simulink model "PreScan_Vissim_Python_0_2_cs_old"  (R2017b)
settings: Solver=ode5  StartTime=0.0  StopTime=inf  FixedStep=1/200  RelTol=1e-3
PreLoadFcn:
  | mbxruntime.callbacks.PreLoadFcn(bdroot);
PostLoadFcn:
  | mbxruntime.callbacks.PostLoadFcn(bdroot);
InitFcn:
  | mbxruntime.callbacks.InitFcn(bdroot);
StartFcn:
  | mbxruntime.callbacks.StartFcn(bdroot);
StopFcn:
  | mbxruntime.callbacks.StopFcn(bdroot);
model workspace (MAT data in the model file):
  mbox_table : struct (value not decoded)
  model_closed = 0
  sim_status = 0
undefined symbols (not defined in the file or in its folder): DiscIntNeverNeededParam, warningInitialVelocity, x0
libraries: simulink x19, simulink_extras x5, dspnetwork x5, PreScanSimulinkLibrary x4, etargetslib x4
(part 4 of 4)

== system PreScan_Vissim_Python_0_2_cs_old/Toyota_Yaris_Hatchback_1/PathFollower_Preview_1/LateralController/CTRL REFERENCES/Find Reference Point (pref0) on Trajectory closest to P0 Point (p0) ==
  In1 : Inport
  In2 : Inport  Port=2
  In3 : Inport  Port=3
  In4 : Inport  Port=4
  eml_find_closest_trajectory_points0 : MATLAB Function  TreatAsAtomicUnit=on
  Out1 : Outport
  Out2 : Outport  Port=2
  wires:
  eml_find_closest_trajectory_points0/2(Actor_traj_angle) -> Out2/1
  eml_find_closest_trajectory_points0/1(Actor_traj_distance) -> Out1/1
  In4/1 -> eml_find_closest_trajectory_points0/4(p0)
  In3/1 -> eml_find_closest_trajectory_points0/3(ActorOffset_Left_Right)
  In2/1 -> eml_find_closest_trajectory_points0/2(TrajOffset_x_y_Y)
  In1/1 -> eml_find_closest_trajectory_points0/1(pvp)

== system PreScan_Vissim_Python_0_2_cs_old/Toyota_Yaris_Hatchback_1/PathFollower_Preview_1/LateralController/SteeringWheelAngle/FirstOrderDynamics ==
  In : Inport
  TimeConstant[s] : Inport  Port=2
  Reset : Inport  Port=3
  x0 : Inport  Port=4
  1|TimeConstant : Product  Inputs=*/  SaturateOnIntegerOverflow=on  InputSameDT=on  OutDataTypeStr=Inherit: Same as first input
  Discrete-Time Integrator : DiscreteIntegrator  ExternalReset=rising  InitialConditionSource=external  InitialCondition=x0  SampleTime=CSSampleTime  ICPrevOutput=DiscIntNeverNeededParam  ICPrevScaledInput=DiscIntNeverNeededParam
  IC : InitialCondition  Value=0
  Saturation : Saturate  UpperLimit=1e300  LowerLimit=0.001
  Sum : Sum  Inputs=-+|  SaturateOnIntegerOverflow=on  InputSameDT=on  OutDataTypeStr=Inherit: Same as first input
  Out : Outport
  wires:
  IC/1 -> Discrete-Time Integrator/3
  In/1 -> Sum/2
  x0/1 -> IC/1
  Reset/1 -> Discrete-Time Integrator/2
  1|TimeConstant/1 -> Discrete-Time Integrator/1
  Sum/1 -> 1|TimeConstant/1
  Saturation/1 -> 1|TimeConstant/2
  TimeConstant[s]/1 -> Saturation/1
  Discrete-Time Integrator/1 -> Out/1, Sum/1

== system PreScan_Vissim_Python_0_2_cs_old/Toyota_Yaris_Hatchback_1/PathFollower_Preview_1/LateralController/SteeringWheelAngle/Sat_Total ==
  In : Inport
  Sat_Limit : Inport  Port=2
  Gain1 : Gain  Gain=-1  SaturateOnIntegerOverflow=on  OutDataTypeStr=Inherit: Same as input  ParamDataTypeStr=Inherit: Same as input
  RelOp_UL : RelationalOperator  RndMeth=Nearest
  RelOp_UL1 : RelationalOperator  Operator=<=  RndMeth=Nearest
  Sum : Sum  Inputs=++|  SaturateOnIntegerOverflow=on
  Switch : Switch  Threshold=0.5  SaturateOnIntegerOverflow=on
  Switch1 : Switch  Threshold=0.5  SaturateOnIntegerOverflow=on
  Sat_Total : Outport
  Sat_Info : Outport  Port=2
  wires:
  Sat_Limit/1 -> Gain1/1, Switch/1, RelOp_UL/2
  RelOp_UL/1 -> Switch/2, Sum/2
  Switch/1 -> RelOp_UL1/1, Switch1/3
  Gain1/1 -> RelOp_UL1/2, Switch1/1
  RelOp_UL1/1 -> Switch1/2, Sum/1
  In/1 -> Switch/3, RelOp_UL/1
  Switch1/1 -> Sat_Total/1
  Sum/1 -> Sat_Info/1

== system PreScan_Vissim_Python_0_2_cs_old/Toyota_Yaris_Hatchback_1/PathFollower_Preview_1/LongitudinalController/If Desired Velocity ~= 0/PID_AWU ==
  e : Inport
  Derivative Gain : Gain  Gain=D  SaturateOnIntegerOverflow=on  OutDataTypeStr=Inherit: Same as input  ParamDataTypeStr=Inherit: Same as input
  Discrete-Time Integrator : DiscreteIntegrator  gainval=1  SampleTime=CSSampleTime  UpperSaturationLimit=100  LowerSaturationLimit=-100  ICPrevOutput=DiscIntNeverNeededParam  ICPrevScaledInput=DiscIntNeverNeededParam
  Filter : DiscreteIntegrator  gainval=1  SampleTime=CSSampleTime  ICPrevOutput=DiscIntNeverNeededParam  ICPrevScaledInput=DiscIntNeverNeededParam
  Integral Gain : Gain  Gain=I  SaturateOnIntegerOverflow=on  OutDataTypeStr=Inherit: Same as input  ParamDataTypeStr=Inherit: Same as input
  Integral Gain1 : Gain  Gain=LongCtrl_AWU  SaturateOnIntegerOverflow=on  OutDataTypeStr=Inherit: Same as input  ParamDataTypeStr=Inherit: Same as input
  Proportional Gain : Gain  Gain=P  SaturateOnIntegerOverflow=on  OutDataTypeStr=Inherit: Same as input  ParamDataTypeStr=Inherit: Same as input
  Saturation : Saturate  UpperLimit=100  LowerLimit=-100
  Sum : Sum  Inputs=+++  SaturateOnIntegerOverflow=on  InputSameDT=on  OutDataTypeStr=Inherit: Same as first input
  Sum1 : Sum  Inputs=|+-  SaturateOnIntegerOverflow=on  InputSameDT=on  OutDataTypeStr=Inherit: Same as first input
  Sum2 : Sum  Inputs=|++  SaturateOnIntegerOverflow=on  InputSameDT=on  OutDataTypeStr=Inherit: Same as first input
  Sum3 : Sum  Inputs=-+|  SaturateOnIntegerOverflow=on  InputSameDT=on  OutDataTypeStr=Inherit: Same as first input
  u : Outport  InitialOutput=0
  wires:
  Integral Gain1/1 -> Sum2/2
  Sum3/1 -> Integral Gain1/1
  Saturation/1 -> Sum3/2, u/1
  Sum2/1 -> Discrete-Time Integrator/1
  Sum1/1 -> Sum/3, Filter/1
  Filter/1 -> Sum1/2
  Derivative Gain/1 -> Sum1/1
  Sum/1 -> Sum3/1, Saturation/1
  e/1 -> Integral Gain/1, Proportional Gain/1, Derivative Gain/1
  Discrete-Time Integrator/1 -> Sum/2
  Proportional Gain/1 -> Sum/1
  Integral Gain/1 -> Sum2/1

== system PreScan_Vissim_Python_0_2_cs_old/Toyota_Yaris_Hatchback_1/Dynamics_Simple/Chassis/Bicycle_model_[XYZ]/X_Motion/Air&RoadResistance ==
  vx_[ms-1] : Inport
  Gain : Gain  Gain=1/p.Rw
  Road & Aerodyn Resistances : Fcn  Expr=p.Rroad + p.Rair*u^2
  Saturation1 : Saturate  UpperLimit=5/15  LowerLimit=-5/15
  Sign : Signum
  "[ms-1] 2 [rads-1]" : Gain  Gain=1/p.Rw  SaturateOnIntegerOverflow=on  OutDataTypeStr=Inherit: Same as input  ParamDataTypeStr=Inherit: Same as input
  signed load1 : Product  SaturateOnIntegerOverflow=on  InputSameDT=on  OutDataTypeStr=Inherit: Same as first input
  Resistance_Force : Outport
  wires:
  signed load1/1 -> Resistance_Force/1  "F_[N]"
  vx_[ms-1]/1 -> Road & Aerodyn Resistances/1, "[ms-1] 2 [rads-1]"/1
  Saturation1/1 -> Sign/1
  "[ms-1] 2 [rads-1]"/1 -> Saturation1/1
  Road & Aerodyn Resistances/1 -> Gain/1  "ResistanceTorque_[Nm]"
  Sign/1 -> signed load1/2  "sign"
  Gain/1 -> signed load1/1  "Resistance Force_[N]"

== system PreScan_Vissim_Python_0_2_cs_old/Toyota_Yaris_Hatchback_1/Dynamics_Simple/Chassis/Bicycle_model_[XYZ]/X_Motion/BrakeSystem ==
  vx_[ms-1] : Inport
  BrakePressure_[bar] : Inport  Port=2
  Gain : Gain  Gain=1/p.Rw
  Saturation : Saturate  UpperLimit=p.PBrakeMax  LowerLimit=0
  Saturation1 : Saturate  UpperLimit=5/15  LowerLimit=-5/15
  Sign : Signum
  "[ms-1] 2 [rads-1]" : Gain  Gain=1/p.Rw  SaturateOnIntegerOverflow=on  OutDataTypeStr=Inherit: Same as input  ParamDataTypeStr=Inherit: Same as input
  braking Q factor : Gain  Gain=p.Qfac  SaturateOnIntegerOverflow=on  OutDataTypeStr=Inherit: Same as input  ParamDataTypeStr=Inherit: Same as input
  signed load1 : Product  SaturateOnIntegerOverflow=on  InputSameDT=on  OutDataTypeStr=Inherit: Same as first input
  BrakeForce : Outport
  BrakeTorqueAbs : Outport  Port=2
  wires:
  braking Q factor/1 -> BrakeTorqueAbs/1, Gain/1
  BrakePressure_[bar]/1 -> Saturation/1
  Saturation/1 -> braking Q factor/1
  vx_[ms-1]/1 -> "[ms-1] 2 [rads-1]"/1
  Saturation1/1 -> Sign/1
  "[ms-1] 2 [rads-1]"/1 -> Saturation1/1
  Sign/1 -> signed load1/2  "sign"
  signed load1/1 -> BrakeForce/1
  Gain/1 -> signed load1/1

== system PreScan_Vissim_Python_0_2_cs_old/Toyota_Yaris_Hatchback_1/Dynamics_Simple/Chassis/Bicycle_model_[XYZ]/X_Motion/Configurable Subsystem ==
  In1 : Inport
  In2 : Inport  Port=2
  In3 : Inport  Port=3
  Integrator : Integrator  ExternalReset=level  InitialConditionSource=external
  Out1 : Outport
  wires:
  In1/1 -> Integrator/1
  In2/1 -> Integrator/2
  In3/1 -> Integrator/3
  Integrator/1 -> Out1/1

== system PreScan_Vissim_Python_0_2_cs_old/Toyota_Yaris_Hatchback_1/Dynamics_Simple/Chassis/Bicycle_model_[XYZ]/X_Motion/Configurable Subsystem1 ==
  In1 : Inport
  Torsional damping : TransferFcn  Denominator=[0.1 1]
  Out1 : Outport
  wires:
  In1/1 -> Torsional damping/1
  Torsional damping/1 -> Out1/1

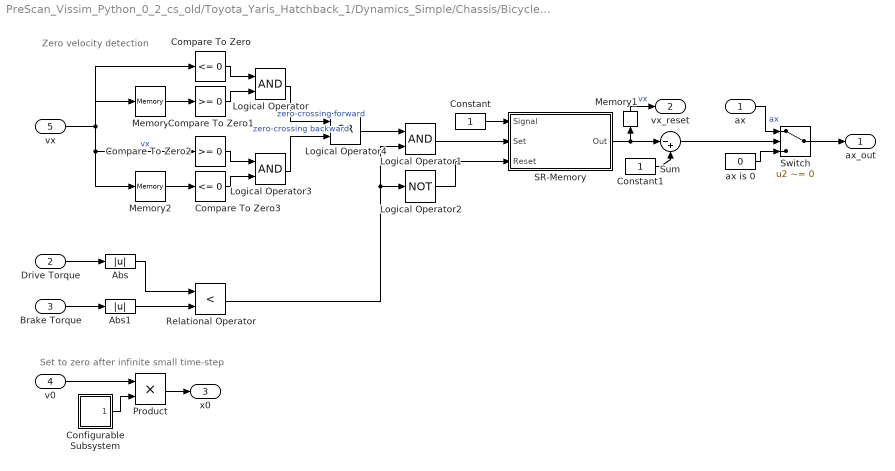
== system PreScan_Vissim_Python_0_2_cs_old/Toyota_Yaris_Hatchback_1/Dynamics_Simple/Chassis/Bicycle_model_[XYZ]/X_Motion/Max RPM and zero- velocity detection ==
  note: Set to zero after infinite small time-step
  note: Zero velocity detection
  ax : Inport
  Drive Torque : Inport  Port=2
  Brake Torque : Inport  Port=3
  v0 : Inport  Port=4
  vx : Inport  Port=5
  Abs : Abs
  Abs1 : Abs
  Compare To Zero : simulink/Logic and Bit Operations/Compare To Zero  relop=<=  OutDataTypeStr=boolean  ZeroCross=off
  Compare To Zero1 : simulink/Logic and Bit Operations/Compare To Zero  relop=>=  OutDataTypeStr=boolean  ZeroCross=off
  Compare To Zero2 : simulink/Logic and Bit Operations/Compare To Zero  relop=>=  OutDataTypeStr=boolean  ZeroCross=off
  Compare To Zero3 : simulink/Logic and Bit Operations/Compare To Zero  relop=<=  OutDataTypeStr=boolean  ZeroCross=off
  Configurable Subsystem : Subsystem  BlockChoice=Step  mask{ComputationMode=ComputationMode}
      mask prompts: ComputationMode "Compuation mode:"
      mask init:
      | SetComputationMode(gcb,ComputationMode);
      settings: AttributesFormatString=%<BlockChoice>  OpenFcn=BringToFront(gcb);  MemberBlocks=Discrete Step,Step
      settings: TemplateBlock=|
      | PreScanSimulinkLibrary/Configurable Subsystems/Step Function/Configurable
      | Subsystem
  Constant : Constant
  Constant1 : Constant
  Logical Operator : Logic  AllPortsSameDT=off  OutDataTypeStr=boolean
  Logical Operator1 : Logic  AllPortsSameDT=off  OutDataTypeStr=boolean
  Logical Operator2 : Logic  Operator=NOT  AllPortsSameDT=off  OutDataTypeStr=boolean
  Logical Operator3 : Logic  AllPortsSameDT=off  OutDataTypeStr=boolean
  Logical Operator4 : Logic  Operator=OR  AllPortsSameDT=off  OutDataTypeStr=boolean
  Memory : Memory
  Memory1 : Memory
  Memory2 : Memory
  Product : Product  RndMeth=Zero
  Relational Operator : RelationalOperator  Operator=<  OutDataTypeStr=boolean  RndMeth=Nearest
  SR-Memory : Subsystem
  Sum : Sum  Inputs=|-+
  Switch : Switch  Criteria=u2 ~= 0  Threshold=0.5
  ax is 0 : Constant  Value=0
  ax_out : Outport
  vx_reset : Outport  Port=2
  x0 : Outport  Port=3
  wires:
  Logical Operator4/1 -> Logical Operator1/1
  vx/1 -> Compare To Zero/1, Compare To Zero2/1, Memory2/1, Memory/1  "vx"
  Memory2/1 -> Compare To Zero3/1
  Compare To Zero2/1 -> Logical Operator3/1
  Compare To Zero3/1 -> Logical Operator3/2
  Logical Operator3/1 -> Logical Operator4/2  "zero-crossing backward"
  Memory/1 -> Compare To Zero1/1
  Compare To Zero/1 -> Logical Operator/1
  Compare To Zero1/1 -> Logical Operator/2
  Logical Operator/1 -> Logical Operator4/1  "zero-crossing forward"
  Abs/1 -> Relational Operator/1
  Abs1/1 -> Relational Operator/2
  Drive Torque/1 -> Abs/1
  Brake Torque/1 -> Abs1/1
  Relational Operator/1 -> Logical Operator1/2, Logical Operator2/1
  Logical Operator1/1 -> SR-Memory/2(Set)
  Constant/1 -> SR-Memory/1(Signal)
  Logical Operator2/1 -> SR-Memory/3(Reset)
  SR-Memory/1(Out) -> Sum/1, Memory1/1
  Switch/1 -> ax_out/1
  Sum/1 -> Switch/2
  ax is 0/1 -> Switch/3
  Constant1/1 -> Sum/2
  v0/1 -> Product/1
  Product/1 -> x0/1
  Configurable Subsystem/1(Out1) -> Product/2
  ax/1 -> Switch/1  "ax"
  Memory1/1 -> vx_reset/1  "vx"

== system PreScan_Vissim_Python_0_2_cs_old/Toyota_Yaris_Hatchback_1/Dynamics_Simple/Chassis/Bicycle_model_[XYZ]/Y & Yaw_Motion/Configurable Subsystem ==
  In1 : Inport
  In2 : Inport  Port=2
  Integrator : Integrator  ExternalReset=level
  Out1 : Outport
  wires:
  In1/1 -> Integrator/1
  In2/1 -> Integrator/2
  Integrator/1 -> Out1/1

== system PreScan_Vissim_Python_0_2_cs_old/Toyota_Yaris_Hatchback_1/Dynamics_Simple/Chassis/Bicycle_model_[XYZ]/Y & Yaw_Motion/Configurable Subsystem1 ==
  In1 : Inport
  Integrator : Integrator
  Out1 : Outport
  wires:
  In1/1 -> Integrator/1
  Integrator/1 -> Out1/1

== system PreScan_Vissim_Python_0_2_cs_old/Toyota_Yaris_Hatchback_1/Dynamics_Simple/Chassis/Bicycle_model_[XYZ]/Y & Yaw_Motion/Configurable Subsystem2 ==
  In1 : Inport
  In2 : Inport  Port=2
  Integrator : Integrator  ExternalReset=level
  Out1 : Outport
  wires:
  In1/1 -> Integrator/1
  In2/1 -> Integrator/2
  Integrator/1 -> Out1/1

== system PreScan_Vissim_Python_0_2_cs_old/Toyota_Yaris_Hatchback_1/Dynamics_Simple/Chassis/Bicycle_model_[XYZ]/Z, Pitch_Motion & Roll_Motion/Configurable Subsystem ==
  In1 : Inport
  Integrator : Integrator  LimitOutput=on  UpperSaturationLimit=5*pi/180  LowerSaturationLimit=-5*pi/180
  Out1 : Outport
  wires:
  In1/1 -> Integrator/1
  Integrator/1 -> Out1/1

== system PreScan_Vissim_Python_0_2_cs_old/Toyota_Yaris_Hatchback_1/Dynamics_Simple/Chassis/Bicycle_model_[XYZ]/Z, Pitch_Motion & Roll_Motion/Configurable Subsystem1 ==
  In1 : Inport
  Integrator : Integrator
  Out1 : Outport
  wires:
  In1/1 -> Integrator/1
  Integrator/1 -> Out1/1

== system PreScan_Vissim_Python_0_2_cs_old/Toyota_Yaris_Hatchback_1/Dynamics_Simple/Chassis/Bicycle_model_[XYZ]/Z, Pitch_Motion & Roll_Motion/Configurable Subsystem2 ==
  In1 : Inport
  Integrator : Integrator
  Out1 : Outport
  wires:
  In1/1 -> Integrator/1
  Integrator/1 -> Out1/1

== system PreScan_Vissim_Python_0_2_cs_old/Toyota_Yaris_Hatchback_1/Dynamics_Simple/Chassis/Bicycle_model_[XYZ]/Z, Pitch_Motion & Roll_Motion/Configurable Subsystem3 ==
  In1 : Inport
  Integrator : Integrator
  Out1 : Outport
  wires:
  In1/1 -> Integrator/1
  Integrator/1 -> Out1/1

== system PreScan_Vissim_Python_0_2_cs_old/Toyota_Yaris_Hatchback_1/Dynamics_Simple/Chassis/Bicycle_model_[XYZ]/Z, Pitch_Motion & Roll_Motion/Configurable Subsystem4 ==
  In1 : Inport
  Integrator : Integrator
  Out1 : Outport
  wires:
  In1/1 -> Integrator/1
  Integrator/1 -> Out1/1

== system PreScan_Vissim_Python_0_2_cs_old/Toyota_Yaris_Hatchback_1/Dynamics_Simple/Chassis/Bicycle_model_[XYZ]/Z, Pitch_Motion & Roll_Motion/Configurable Subsystem5 ==
  In1 : Inport
  Integrator : Integrator
  Out1 : Outport
  wires:
  In1/1 -> Integrator/1
  Integrator/1 -> Out1/1

== system PreScan_Vissim_Python_0_2_cs_old/Toyota_Yaris_Hatchback_1/Dynamics_Simple/Chassis/Bicycle_model_[XYZ]/Z, Pitch_Motion & Roll_Motion/Configurable Subsystem9 ==
  In1 : Inport
  Derivative : Derivative
  Out1 : Outport
  wires:
  In1/1 -> Derivative/1
  Derivative/1 -> Out1/1

== system PreScan_Vissim_Python_0_2_cs_old/Toyota_Yaris_Hatchback_1/Dynamics_Simple/Chassis/FrontTyre/AlphaFront/Enabled Subsystem ==
  In : Inport
  Enable : EnablePort  PropagateVarSize=During execution
  AlphaFront : Fcn  Expr=-atan( (u(2)+u(3)*p.a)/u(1) )
  Alpha : Outport  OutputWhenDisabled=reset  InitialOutput=[0]
  wires:
  AlphaFront/1 -> Alpha/1
  In/1 -> AlphaFront/1

== system PreScan_Vissim_Python_0_2_cs_old/Toyota_Yaris_Hatchback_1/Dynamics_Simple/Chassis/RearTyre/AlphaRear/Enabled Subsystem ==
  In : Inport
  Enable : EnablePort  PropagateVarSize=During execution
  AlphaRear : Fcn  Expr=-atan( (u(2)-u(3)*p.b)/u(1) )
  Alpha : Outport  OutputWhenDisabled=reset  InitialOutput=[0]
  wires:
  AlphaRear/1 -> Alpha/1
  In/1 -> AlphaRear/1

== system PreScan_Vissim_Python_0_2_cs_old/Toyota_Yaris_Hatchback_1/Dynamics_Simple/Chassis/Bicycle_model_[XYZ]/X_Motion/Max RPM and zero- velocity detection/Configurable Subsystem ==
  Step : Step  Time=0.0001  Before=1  After=0  SampleTime=0
  Out1 : Outport
  wires:
  Step/1 -> Out1/1

== system PreScan_Vissim_Python_0_2_cs_old/Toyota_Yaris_Hatchback_1/Dynamics_Simple/Chassis/Bicycle_model_[XYZ]/X_Motion/Max RPM and zero- velocity detection/SR-Memory ==
  Signal : Inport
  Set : Inport  Port=2
  Reset : Inport  Port=3
  Constant : Constant  Value=0
  Detect Rise Positive : simulink/Logic and Bit Operations/Detect Rise Positive  vinit=0  OutDataTypeStr=uint8
  Detect Rise Positive1 : simulink/Logic and Bit Operations/Detect Rise Positive  vinit=0  OutDataTypeStr=uint8
  Manual Switch : ManualSwitch
  Manual Switch1 : ManualSwitch
  Switch : Switch  Criteria=u2 ~= 0
  Switch1 : Switch  Criteria=u2 ~= 0
  Unit Delay : UnitDelay  SampleTime=-1
  Out : Outport
  wires:
  Constant/1 -> Switch1/1
  Switch/1 -> Switch1/3
  Switch1/1 -> Unit Delay/1, Out/1
  Manual Switch1/1 -> Switch1/2
  Reset/1 -> Manual Switch1/2, Detect Rise Positive1/1
  Detect Rise Positive1/1 -> Manual Switch1/1
  Signal/1 -> Switch/1
  Unit Delay/1 -> Switch/3
  Set/1 -> Detect Rise Positive/1, Manual Switch/2
  Detect Rise Positive/1 -> Manual Switch/1
  Manual Switch/1 -> Switch/2

== matlab function PreScan_Vissim_Python_0_2_cs_old/Toyota_Yaris_Hatchback_1/PathFollower_Preview_1/LateralController/CTRL REFERENCES/Calculate Lateral Error/eml_find_10k_lateral_error_points ==
  settings: updateMethod=DISCRETE
  data: pvp input size=2; dist_psvehicle output size=10; TrajOffset_x_y_Y input size=3; ActorOffset_Left_Right input; p0 input size=2; PreviewDistance input size=10; Traj_x parameter; Traj_y parameter; Traj_t parameter; Traj_v parameter; RefreshCounter parameter
function dist_psvehicle  = eml_find_10k_lateral_error_points(pvp,TrajOffset_x_y_Y,ActorOffset_Left_Right,p0,PreviewDistance,Traj_x,Traj_y,Traj_t,Traj_v,RefreshCounter)

dist_psvehicle = emlfcn_find_10k_lateral_error_points(pvp,TrajOffset_x_y_Y,ActorOffset_Left_Right,p0,PreviewDistance,Traj_x,Traj_y,Traj_t,Traj_v,RefreshCounter);

% end function

== matlab function PreScan_Vissim_Python_0_2_cs_old/Toyota_Yaris_Hatchback_1/MATLAB Function1 ==
  data: u input; y output
function y = fcn(u)

    u(1)=0;
    u(2)=0;

y = u;

== matlab function PreScan_Vissim_Python_0_2_cs_old/Toyota_Yaris_Hatchback_1/PathFollower_Preview_1/LateralController/CTRL REFERENCES/Find Reference Point (pref0) on Trajectory closest to P0 Point (p0)/eml_find_closest_trajectory_points0 ==
  data: pvp input size=2; Actor_traj_distance output; TrajOffset_x_y_Y input size=3; ActorOffset_Left_Right input; p0 input size=3; Traj_x parameter; Traj_y parameter; Actor_traj_angle output; RefreshCounter parameter
function [Actor_traj_distance,Actor_traj_angle]  = eml_find_closest_trajectory_points0(pvp,TrajOffset_x_y_Y,ActorOffset_Left_Right,p0,Traj_x,Traj_y,RefreshCounter)

[Actor_traj_distance,Actor_traj_angle]  = emlfcn_find_closest_trajectory_points0(pvp,TrajOffset_x_y_Y,ActorOffset_Left_Right,p0,Traj_x,Traj_y,RefreshCounter);

% end function

== matlab function PreScan_Vissim_Python_0_2_cs_old/Toyota_Yaris_Hatchback_1/MATLAB Function2 ==
  data: u input; y output
function y = fcn(u)

y = u(1);

== matlab function PreScan_Vissim_Python_0_2_cs_old/Toyota_Yaris_Hatchback_1/PathFollower_Preview_1/LateralController/Calculate delta steering error/eml_delta_steering_error ==
  data: v_x_vehicle input; v_x_vehicle_Min input; t_Preview_LatCtrl input; delta_steeringwheeltotal output; v_y_vehicle input; yawrate_vehicle input; CorneringStiffness_Tyres_Front input; CorneringStiffness_Tyres_Rear input; m_vehicle_total input; inertia_z_vehicle_total input; e_Lat input size=10; Pos_x_CoG_Vehicle input; wheelbase input; RefreshCounter parameter
function delta_steeringwheeltotal = eml_delta_steering_error(v_x_vehicle,v_x_vehicle_Min,t_Preview_LatCtrl,v_y_vehicle,yawrate_vehicle,CorneringStiffness_Tyres_Front,CorneringStiffness_Tyres_Rear,m_vehicle_total,inertia_z_vehicle_total,e_Lat,Pos_x_CoG_Vehicle,wheelbase,RefreshCounter)

delta_steeringwheeltotal = emlfcn_delta_steering_error(v_x_vehicle,v_x_vehicle_Min,t_Preview_LatCtrl,v_y_vehicle,yawrate_vehicle,CorneringStiffness_Tyres_Front,CorneringStiffness_Tyres_Rear,m_vehicle_total,inertia_z_vehicle_total,e_Lat,Pos_x_CoG_Vehicle,wheelbase,RefreshCounter);

% end function

== matlab function PreScan_Vissim_Python_0_2_cs_old/Toyota_Yaris_Hatchback_1/MATLAB Function ==
  data: u input; y output
function y = fcn(u)

y = u(1);
%pause(1);

== matlab function PreScan_Vissim_Python_0_2_cs_old/Toyota_Yaris_Hatchback_1/MATLAB Function7 ==
  data: IDs input; range input; azimuth input; send_data output; vel input; state input; if_collide input; Collid_1 input; Collid_2 input
function send_data = fcn(IDs,range,azimuth ,vel ,state, if_collide,Collid_1,Collid_2)
coder.extrinsic('mat2str','disp','num2str','bdroot','get_param');


Number_data=10;
pt = 10;


t = num2str(round(get_param(bdroot,'SimulationTime'),pt),['%0' num2str(pt) '.2f ']);
% t = num2str(2.2,['%0.' num2str(pt) 'f ']);

To_add=['{"Time":"' t '", '];


for i=1:Number_data
    Id_name=num2str(i,['%0' num2str(3) '.f ']);
    Id_Colide=num2str(IDs(i),['%0' num2str(pt) '.f ']);
    Ra_Colide=num2str(range(i),['%0' num2str(pt) '.2f ']);
    az_Colide=num2str(azimuth(i),['%0' num2str(pt) '.2f ']);
    Ve_Colide=num2str(vel(i),['%0' num2str(pt) '.2f ']);
    
    
    To_add=[To_add '"Id' Id_name '":"' Id_Colide '", ' ...
                   '"Range' Id_name '":"' Ra_Colide '", ' ...
                   '"Azimuth' Id_name '":"' az_Colide '"' ...
                   '"Velocity' Id_name '":"' Ve_Colide '", '] ;
   if i<Number_data
       To_add=[To_add ', '];
   end
end

To_add=[To_add ', ']

pInput = 15;
pt = 10;
% % % % % % % % % % % % % % % % % 
p = pInput + 7;
state(isnan(state)) = 0;
u = zeros(9,p);
m = num2str([state(:);-1], ['% .' num2str(pInput) 'e ']);
sss = 1:p;
u(1,sss) = m(1,sss);    
u(2,sss) = m(2,sss);
u(3,sss) = m(3,sss);
u(4,sss) = m(4,sss);



To_add=[To_add '"Position":{"x":' u(1,:) ',"y":' u(2,:) '},' ...
        '"Velocity":' u(3,:) ',' ...
        '"Heading":' u(3,:) ',' ...
        '"Reward":' u(4,:) ',' ];

% To_add=[To_add '"Position":{"x":' u(1,:) ',"y":' u(2,:) '},' ...
%         '"Velocity":' u(3,:) ',' ...
%         '"Heading":' u(3,:) ',' ...
%         '"Reward":' u(4,:) '}' ];
    
    
if_collide_s=num2str((if_collide),['%0' num2str(pt) '.f ']);
Collid_1_s=num2str(Collid_1,['%0' num2str(pt) '.f ']);
Collid_2_s=num2str(Collid_2,['%0' num2str(pt) '.f ']);

To_add=[To_add '"if_collide":"' if_collide_s '",'  ...
                '"Collid_1":"' Collid_1_s '",'  ...
                '"Collid_2":"' Collid_2_s '"}'];


len=1102;
send_data = uint8(32*ones(len,1));

send_data = uint8(To_add);
send_data = uint8(send_data);

== matlab function PreScan_Vissim_Python_0_2_cs_old/Toyota_Yaris_Hatchback_1/MATLAB Function3 ==
  data: u input; y output
function y = fcn(u)

y = u(1);

== matlab function PreScan_Vissim_Python_0_2_cs_old/Toyota_Yaris_Hatchback_1/MATLAB Function4 ==
  data: u input; y output
function y = fcn(u)

y = u(1);

== matlab function PreScan_Vissim_Python_0_2_cs_old/Toyota_Yaris_Hatchback_1/MATLAB Function5 ==
  data: u input; y output
function y = fcn(u)

y = u(1);

== matlab function PreScan_Vissim_Python_0_2_cs_old/Toyota_Yaris_Hatchback_1/MATLABFunction6 ==
  data: x input; y output
function y = fcn(x)

coder.extrinsic('set_param')
%coder.extrinsic('bdroot')
coder.extrinsic('sim')
  
y = 0;

if (x>601) 
    set_param('PreScan_Vissim_Python_0_cs', 'SimulationCommand', 'stop');
    y = 1;
end
